simulink model "Model"  (R2022a)
settings: Solver=VariableStepAuto  StartTime=0.0  StopTime=8400  RelTol=1e-3
values from neighbouring files (symbols this model uses):
  C1 = 100    [script.m]
  C2 = 60    [script.m]
  R12 = ((R1*R2)/(R1+R2))    (= 5)    [script.m]
  R2 = 10    [script.m]
  R23 = ((R2*R3)/(R2+R3))    (= 5)    [script.m]
  Theta_A = 293.15    [script.m]
settings Model: Creator=97450  LastModifiedBy=zaidd

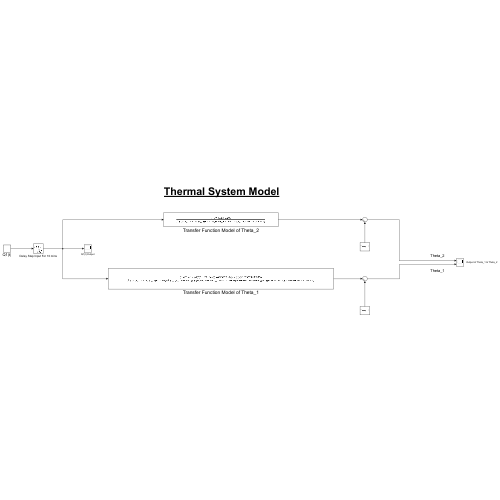
[thumbnail: Simulink's stored preview of the top-level diagram]
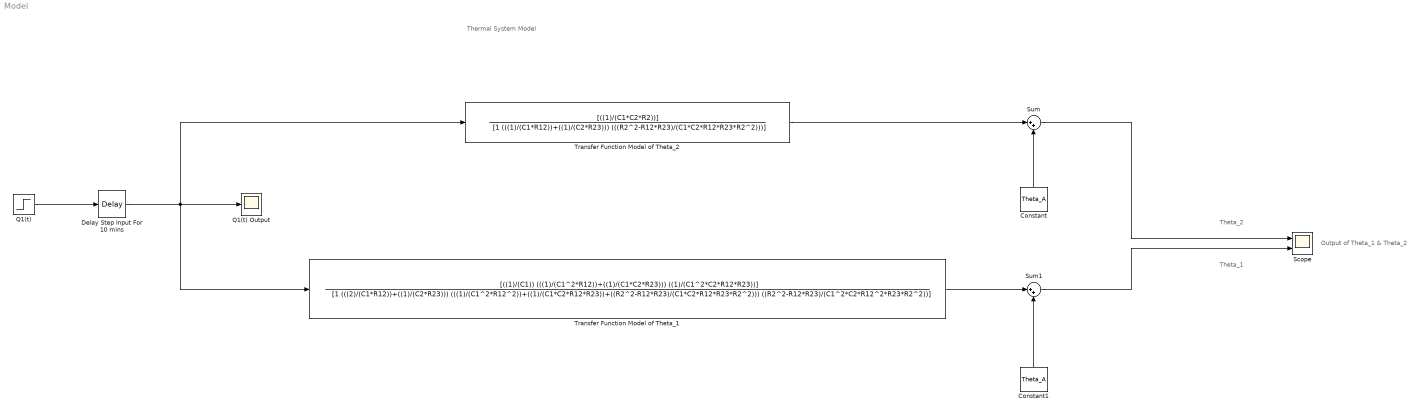
== system Model ==
  note: Output of Theta_1 & Theta_2
  note: Thermal System Model
  note: Theta_2
  note: Theta_1
  Constant : Constant  Value=Theta_A
  Constant1 : Constant  Value=Theta_A
  Delay Step Input For 10 mins : TransportDelay  DelayTime=600
  Q1(t) : Step  After=3  SampleTime=0
  Q1(t) Output : Scope
  Scope : Scope  NumInputPorts=2
  Sum : Sum  Inputs=|++
  Sum1 : Sum  Inputs=|++
  Transfer Function Model of Theta_1 : TransferFcn  Numerator=[((1)/(C1)) (((1)/(C1^2*R12))+((1)/(C1*C2*R23))) ((1)/(C1^2*C2*R12*R23))]  Denominator=[1 (((2)/(C1*R12))+((1)/(C2*R23))) (((1)/(C1^2*R12^2))+((1)/(C1*C2*R12*R23))+((R2^2-R12*R23)/(C1*C2*R12*R23*R2^2))) ((R2^2-R12*R23)/(C1^2*C2*R12^2*R23*R2^2))]
  Transfer Function Model of Theta_2 : TransferFcn  Numerator=[((1)/(C1*C2*R2))]  Denominator=[1 (((1)/(C1*R12))+((1)/(C2*R23))) (((R2^2-R12*R23)/(C1*C2*R12*R23*R2^2)))]
  wires:
  Constant/1 -> Sum/2
  Transfer Function Model of Theta_2/1 -> Sum/1
  Transfer Function Model of Theta_1/1 -> Sum1/1
  Constant1/1 -> Sum1/2
  Q1(t)/1 -> Delay Step Input For 10 mins/1
  Delay Step Input For 10 mins/1 -> Q1(t) Output/1, Transfer Function Model of Theta_2/1, Transfer Function Model of Theta_1/1
  Sum1/1 -> Scope/2
  Sum/1 -> Scope/1
